simulink model "safe_control"  (R2025b)
settings: Solver=FixedStepAuto  StartTime=0.0  StopTime=t_end  FixedStep=dt  RelTol=1e-3
values from neighbouring files (symbols this model uses):
  p_r = [-3 2.5]    [data0.mat]    (also in data1.mat; data10.mat)
undefined symbols (not defined in the file or in its folder): delta_obs, dt, ganmm, kp, p_init, p_obs
libraries: slctrl_constraint x1
settings Model: Creator=yamauchi  LastModifiedBy=tanabe

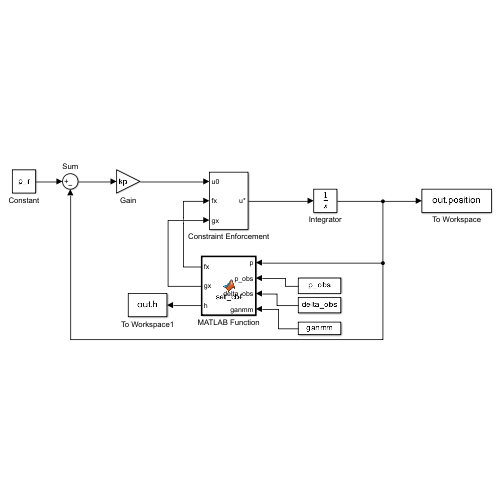
[thumbnail: Simulink's stored preview of the top-level diagram]
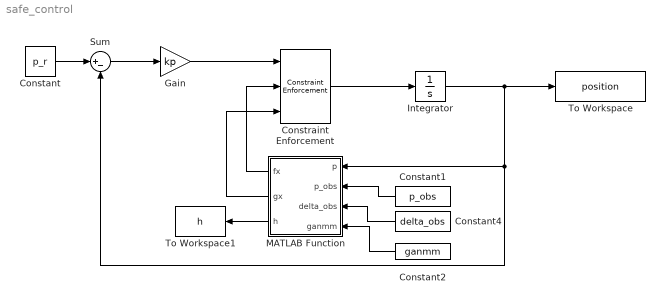
== system safe_control ==
  Constant : Constant  Value=p_r
  Constant1 : Constant  Value=p_obs
  Constant2 : Constant  Value=ganmm
  Constant4 : Constant  Value=delta_obs
  Constraint Enforcement : slctrl_constraint/Constraint Enforcement  nc=1  nu=2  c=0  external_c=off  external_umax=off  external_umin=off  Ts=dt  maxiter=200  tol=1e-6  output_exitflag=off  relax_c=off  relax_u=off
      settings: LibrarySourceBlock=slctrlblks/Constraint Control/Constraint Enforcement
  Gain : Gain  Gain=kp
  Integrator : Integrator  InitialCondition=p_init
  MATLAB Function : MATLAB Function  TreatAsAtomicUnit=on
  Sum : Sum  Inputs=|+-
  To Workspace : ToWorkspace  VariableName=position  SampleTime=-1
      settings: Save2DSignal=2-D array (concatenate along first dimension)
  To Workspace1 : ToWorkspace  VariableName=h  SampleTime=-1
      settings: Save2DSignal=2-D array (concatenate along first dimension)
  wires:
  Gain/1 -> Constraint Enforcement/1
  Constant/1 -> Sum/1
  Sum/1 -> Gain/1
  Integrator/1 -> To Workspace/1, Sum/2, MATLAB Function/1(p)
  Constant4/1 -> MATLAB Function/3(delta_obs)
  Constant1/1 -> MATLAB Function/2(p_obs)
  MATLAB Function/1(fx) -> Constraint Enforcement/2
  MATLAB Function/2(gx) -> Constraint Enforcement/3
  Constraint Enforcement/1 -> Integrator/1
  MATLAB Function/3(h) -> To Workspace1/1
  Constant2/1 -> MATLAB Function/4(ganmm)

== matlab function safe_control/MATLAB Function ==
  data: p input; fx output; p_obs input; delta_obs input; gx output; h output; ganmm input
function [fx, gx, h] = set_cbf(p, p_obs, delta_obs,ganmm)

h = norm(p-p_obs)^2 - delta_obs^2;
fx = -ganmm*h;
gx = 2*(p_obs-p)';
